simulink model "PTC_MBDS_Modulo_Sample"  (R2013a)
settings: Solver=FixedStepDiscrete  StartTime=0.0  StopTime=100  FixedStep=Auto  RelTol=1e-3
libraries: PTC_MBDS_LIB x2, simulink_extras x1
settings Model: Creator=uidl7367  LastModifiedBy=sundeep.tuteja
settings DataIOCC: SignalLoggingSaveFormat=ModelDataLogs
settings OptimizationCC: ExpressionDepthLimit=2147483647  InitFltsAndDblsToZero=on
settings DebuggingCC: SaveWithParameterizedLinksMsg=none  SignalResolutionControl=TryResolveAllWithWarning  SolverPrmCheckMsg=none  InheritedTsInSrcMsg=none  MultiTaskDSMMsg=warning  MultiTaskCondExecSysMsg=none  ParameterPrecisionLossMsg=none  FcnCallInpInsideContextMsg=UseLocalSettings  StrictBusMsg=Warning
settings RTWCC: IncludeERTFirstTime=on
settings GRTTargetCC: TargetFcnLib=ansi_tfl_tmw.mat  CombineOutputUpdateFcns=off  GRTInterface=on

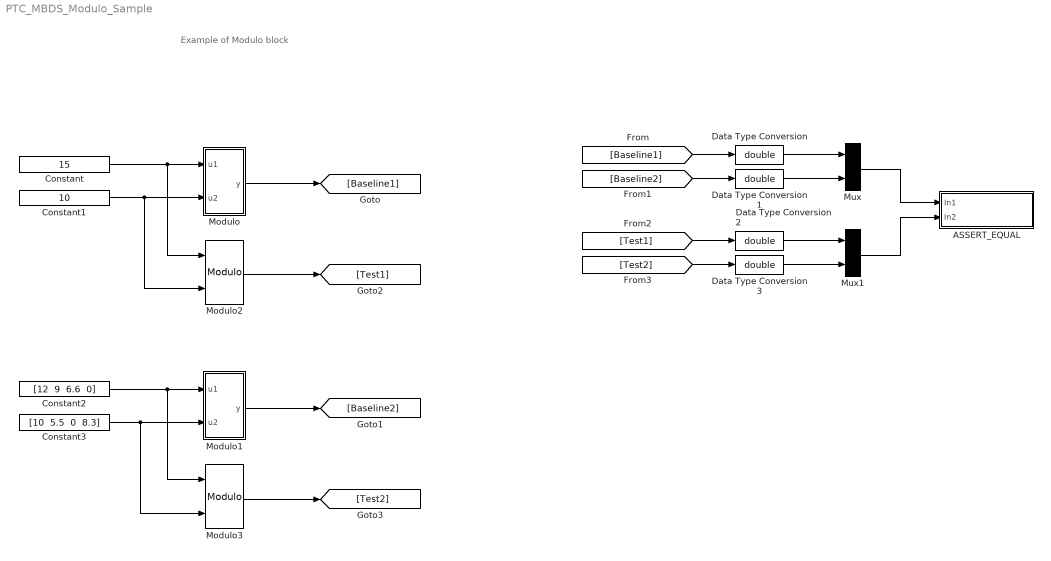
== system PTC_MBDS_Modulo_Sample ==
  note: Example of Modulo block
  ASSERT_EQUAL : Subsystem
  Constant : Constant  InitFcn=|  Value=15  OutDataTypeStr=uint8
      | if(exist('MBDS_BlockCallback', 'file'))
      |    MBDS_BlockCallback('Update', gcb);  
      | end
  Constant1 : Constant  InitFcn=|  Value=10  OutDataTypeStr=uint8
      | if(exist('MBDS_BlockCallback', 'file'))
      |    MBDS_BlockCallback('Update', gcb);  
      | end
  Constant2 : Constant  InitFcn=|  Value="[12  9  6.6  0]"  OutDataTypeStr=uint16
      | if(exist('MBDS_BlockCallback', 'file'))
      |    MBDS_BlockCallback('Update', gcb);  
      | end
  Constant3 : Constant  InitFcn=|  Value="[10  5.5  0  8.3]"  OutDataTypeStr=uint16
      | if(exist('MBDS_BlockCallback', 'file'))
      |    MBDS_BlockCallback('Update', gcb);  
      | end
  Data Type Conversion{,1..3} (4 alike) : DataTypeConversion  OutDataTypeStr=double
  Modulo : Subsystem  InitFcn=|  mask(Modulo){MBDS_LibraryBlock=on, MBDS_BlockVersion=05.40}
      | if(exist('MBDS_BlockCallback', 'file'))
      |    MBDS_BlockCallback('Update', gcb);
      | end
      mask prompts: MBDS_LibraryBlock "MBDS library block"; MBDS_BlockVersion "Block version:"
      mask help: Modulus after division
      mask init:
      | if(exist('MBDS_BlockCallback', 'file'))
      |    MBDS_BlockCallback('Init', gcb);
      | else
      |    % Disable all mask parameters
      |    MaskEnables = get_param(gcb, 'MaskEnables');
      |    for k = [1:length(MaskEnables)]
      |       MaskEnables{k} = 'off';
      |    end
      |    if(~isequal(MaskEnables, get_param(gcb, 'MaskEnables')))
      |       set_param(gcb, 'MaskEnables', MaskEnables);
      |    end
      | end
      mask Help: eval(['open([workdir(''library_dir:''),''\Blockset\help\'',get_param(gcb,''MaskType''),''.html''])'])
      mask Display:
      | % Show icon or block text
      | disp('mod');
  Modulo1 : Subsystem  InitFcn=|  mask(Modulo){MBDS_LibraryBlock=on, MBDS_BlockVersion=05.40}
      | if(exist('MBDS_BlockCallback', 'file'))
      |    MBDS_BlockCallback('Update', gcb);
      | end
      mask prompts: MBDS_LibraryBlock "MBDS library block"; MBDS_BlockVersion "Block version:"
      mask help: Modulus after division
      mask init: same as PTC_MBDS_Modulo_Sample/Modulo
      mask Help: eval(['open([workdir(''library_dir:''),''\Blockset\help\'',get_param(gcb,''MaskType''),''.html''])'])
      mask Display:
      | % Show icon or block text
      | disp('mod');
  Modulo2 : PTC_MBDS_LIB/MBDS Standard Library/Basic Operations/Math Operations/Modulo  PTC_BlockType=PTC_MBDS_Modulo  PTC_MBDS_BlockVersion=5.32
  Modulo3 : PTC_MBDS_LIB/MBDS Standard Library/Basic Operations/Math Operations/Modulo  PTC_BlockType=PTC_MBDS_Modulo  PTC_MBDS_BlockVersion=5.32
  Mux : Mux  Inputs=2
  Mux1 : Mux  Inputs=2
  wires:
  Constant/1 -> Modulo/1(u1), Modulo2/1
  Constant1/1 -> Modulo/2(u2), Modulo2/2
  Modulo/1(y) -> [Baseline1]
  Constant2/1 -> Modulo1/1(u1), Modulo3/1
  Constant3/1 -> Modulo1/2(u2), Modulo3/2
  Modulo1/1(y) -> [Baseline2]
  Modulo2/1 -> [Test1]
  Modulo3/1 -> [Test2]
  Mux/1 -> ASSERT_EQUAL/1(In1)
  [Baseline1] -> Data Type Conversion/1
  [Baseline2] -> Data Type Conversion1/1
  [Test2] -> Data Type Conversion3/1
  [Test1] -> Data Type Conversion2/1
  Data Type Conversion/1 -> Mux/1
  Data Type Conversion1/1 -> Mux/2
  Data Type Conversion2/1 -> Mux1/1
  Data Type Conversion3/1 -> Mux1/2
  Mux1/1 -> ASSERT_EQUAL/2(In2)

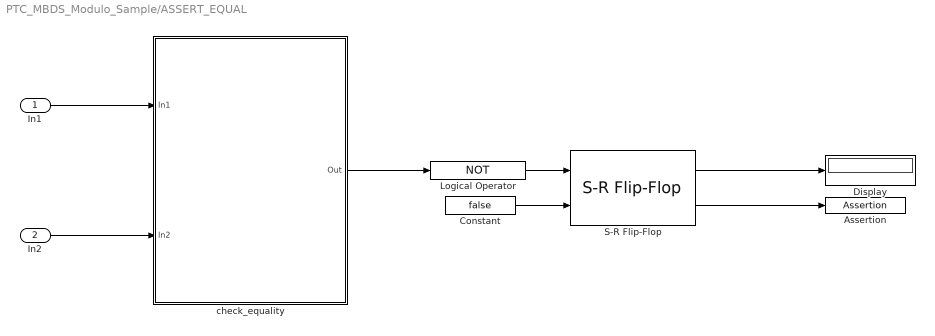
== system PTC_MBDS_Modulo_Sample/ASSERT_EQUAL ==
  In1 : Inport
  In2 : Inport  Port=2
  Assertion : Assertion
  Constant : Constant  Value=false
  Display : Display
  Logical Operator : Logic  Operator=NOT  AllPortsSameDT=off  OutDataTypeStr=boolean
  S-R Flip-Flop : simulink_extras/Flip Flops/S-R Flip-Flop  initial_condition=0
  check_equality : MATLAB Function  TreatAsAtomicUnit=on
  wires:
  S-R Flip-Flop/1 -> Display/1
  check_equality/1(Out) -> Logical Operator/1
  Constant/1 -> S-R Flip-Flop/2
  S-R Flip-Flop/2 -> Assertion/1
  In2/1 -> check_equality/2(In2)
  In1/1 -> check_equality/1(In1)
  Logical Operator/1 -> S-R Flip-Flop/1

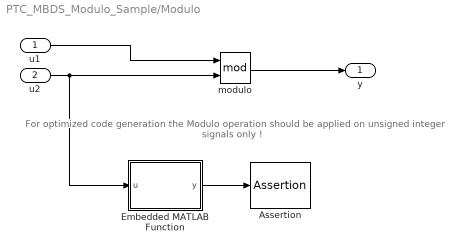
== system PTC_MBDS_Modulo_Sample/Modulo ==
  note: For optimized code generation
      | the Modulo operation should be applied
      |  on unsigned integer signals only !
  u1 : Inport
  u2 : Inport  Port=2
  Assertion : Assertion  AssertionFailFcn=error('Invalid data types used for modulo operation. Apply unsigned integer signals only.')
  Embedded MATLAB Function : MATLAB Function  TreatAsAtomicUnit=on
  modulo : Math  Operator=mod
  y : Outport
  wires:
  Embedded MATLAB Function/1(y) -> Assertion/1
  u2/1 -> modulo/2, Embedded MATLAB Function/1(u)
  u1/1 -> modulo/1
  modulo/1 -> y/1

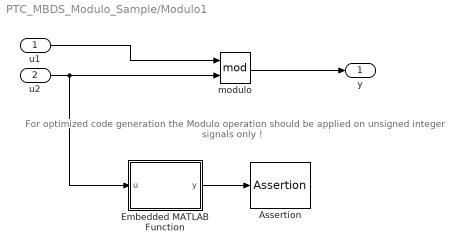
== system PTC_MBDS_Modulo_Sample/Modulo1 ==
  note: For optimized code generation
      | the Modulo operation should be applied
      |  on unsigned integer signals only !
  u1 : Inport
  u2 : Inport  Port=2
  Assertion : Assertion  AssertionFailFcn=error('Invalid data types used for modulo operation. Apply unsigned integer signals only.')
  Embedded MATLAB Function : MATLAB Function  TreatAsAtomicUnit=on
  modulo : Math  Operator=mod
  y : Outport
  wires:
  modulo/1 -> y/1
  u1/1 -> modulo/1
  u2/1 -> Embedded MATLAB Function/1(u), modulo/2
  Embedded MATLAB Function/1(y) -> Assertion/1

== matlab function PTC_MBDS_Modulo_Sample/Modulo1/Embedded MATLAB Function ==
  data: u input; y output
function y = CheckType(u)

% Check for unsigned data types
if(isa(u,'uint8') || isa(u,'uint16') || isa(u,'uint32'))
   y = true;
else   
   y = false;
end

== matlab function PTC_MBDS_Modulo_Sample/Modulo/Embedded MATLAB Function ==
  data: u input; y output
function y = CheckType(u)

% Check for unsigned data types
if(isa(u,'uint8') || isa(u,'uint16') || isa(u,'uint32'))
   y = true;
else   
   y = false;
end

== matlab function PTC_MBDS_Modulo_Sample/ASSERT_EQUAL/check_equality ==
  data: In1 input; Out output; In2 input
function Out = check_equality(In1, In2)
%#codegen

Out = isequaln(In1, In2);

end
